simulink model "comprez"  (R2021b)
settings: Solver=VariableStepAuto  StartTime=0.0  StopTime=220  RelTol=1e-3
values from neighbouring files (symbols this model uses):
  AirDensity_kgpm3 = 1.225    [vehicle_controller.mat]
  BatteryCapacity_Wh = 83    [vehicle_controller.mat]
  BatteryInitialEnergy = 58.1    [vehicle_controller.mat]
  BatteryMaxVoltage_V = 96    [vehicle_controller.mat]
  BatteryVoltageCoefficient_x = [0 0.1 0.2 0.3 0.4 0.5 0.6 0.7 0.8 0.9 1]    [vehicle_controller.mat]
  BatteryVoltageCoefficient_y = [0.833333333333 0.85 0.866666666667 0.883333333333 0.9 0.916666666667 0.933333333333 0.95 0.966666666667 0.983333333333 1]    [vehicle_controller.mat]
  BodyInitialSpeed_mps = 0    [vehicle_controller.mat]
  BodyMass_kg = 900    [vehicle_controller.mat]
  CombustionEngineMaxTorque_Nm = 100    [vehicle_controller.mat]
  DragArea_m2 = 4.5    [vehicle_controller.mat]
  DragCoeficient_1 = 0.4    [vehicle_controller.mat]
  FrictionCoefficient_Nsprad = 0.01    [vehicle_controller.mat]
  GearboxRatio_0_1 = 3    [vehicle_controller.mat]
  Ke = 0.1178    [vehicle_controller.mat]
  Kt = 0.668    [vehicle_controller.mat]
  L = looptransfer.Lo    [H_infinity_control_design.m]    (also in LoopShaping.m = G*K; Vehicle_Car_Controller.m = P * C)
  R = 0.141176    [vehicle_controller.mat]
  WheelDiameter_m = 0.5    [vehicle_controller.mat]
undefined symbols (not defined in the file or in its folder): K
libraries: simulink x10, simulink_extras x3, neural x1
settings Model: Creator=beni  LastModifiedBy=beni

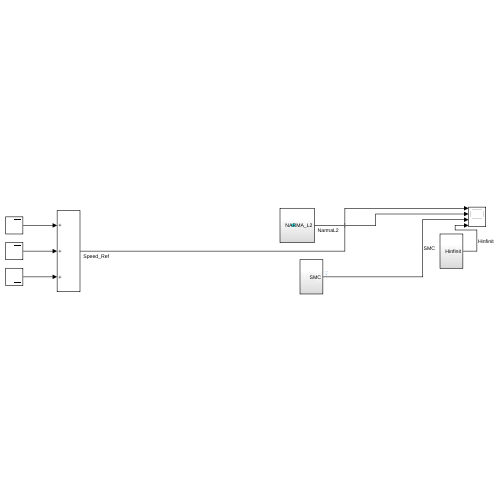
[thumbnail: Simulink's stored preview of the top-level diagram]
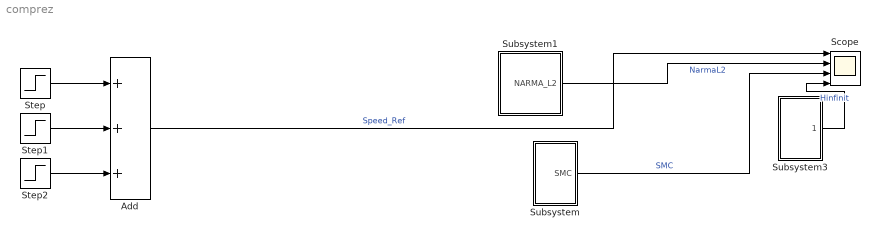
== system comprez ==
  Add : Sum  Inputs=+++
  Scope : Scope  NumInputPorts=4
  Step : Step  After=63  SampleTime=0
  Step1 : Step  Time=100  After=75  SampleTime=0
  Step2 : Step  Time=150  After=-20  SampleTime=0
  Subsystem : Subsystem
  Subsystem1 : Subsystem
  Subsystem3 : Subsystem
  wires:
  Subsystem1/1(NARMA_L2) -> Scope/2  "NarmaL2"
  Subsystem/1(SMC) -> Scope/3  "SMC"
  Subsystem3/1(Hinfinit) -> Scope/4  "Hinfinit"
  Step/1 -> Add/1
  Step2/1 -> Add/3
  Step1/1 -> Add/2
  Add/1 -> Scope/1  "Speed_Ref"

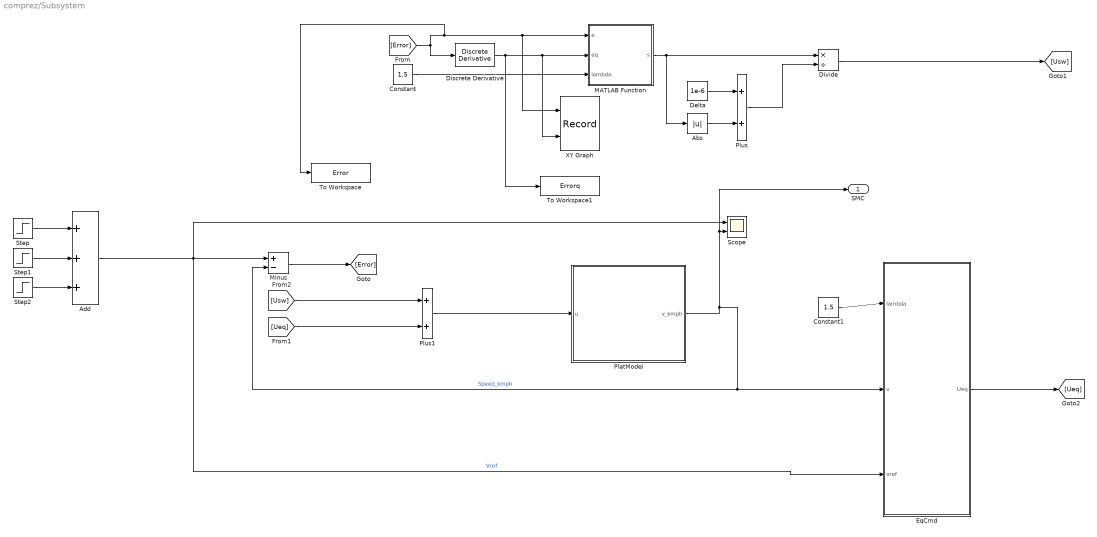
== system comprez/Subsystem ==
  Abs : Abs
  Add : Sum  Inputs=+++
  Constant : Constant  Value=1.5
  Constant1 : Constant  Value=1.5
  Delta : Constant  Value=1e-6
  Discrete Derivative : simulink/Discrete/Discrete Derivative  gainval=1.0  ICPrevScaledInput=0.0  OutMin=[]  OutMax=[]  OutDataType=fixdt(1, 16)  OutScaling=2^-10  DoSatur=off
  Divide : Product  Inputs=*/
  EqCmd : Subsystem
  MATLAB Function : MATLAB Function  TreatAsAtomicUnit=on
  Minus : Sum  Inputs=+-
  PlatModel : Subsystem
  Plus : Sum
  Plus1 : Sum
  Scope : Scope  NumInputPorts=2
  Step : Step  After=63  SampleTime=0
  Step1 : Step  Time=100  After=75  SampleTime=0
  Step2 : Step  Time=150  After=-20  SampleTime=0
  To Workspace : ToWorkspace  VariableName=Error  SampleTime=-1
  To Workspace1 : ToWorkspace  VariableName=Errorq  SampleTime=-1
  XY Graph : Record  FileSettingsInternal="{\"entries\":[{\"content\":{\"excelSettings\":{\"content\":{},\"type\":\"Streamout.ExcelSettings\"}},\"type\":\"Streamout.FileSettingStorage\",\"uuid\":\"431da7f9-c04b-4948-b4ed-e4a663989407\"}],\"packageUris\":[\"http://schema.mathworks.com/mf0/streamout_blocks/R2020a\"],\"version\":\"1.0\"}"  Layout=[1 1]  SignalsInternal="{\"entries\":[{\"content\":{\"signals\":[{\"content\":{\"blockPath\":[\"untitled/Subsystem/XY Graph\"],\"channel\":[],\"dimensions\":[1],\"domain\":\"untitled/Subsystem/XY Graph\",\"lineColor\":\"#77ac30\",\"plots\":[],\"port\":1,\"sid\":[\"\"],\"signalID\":461,\"signalName\":\"From\"},\"type\":\"RecordBlkView.Signal\",\"uuid\":\"f59c2270-2e51-4f55-abe7-1d4243515257\"},{\"content\":{\"blockPath\":[\"untitled/Subsystem/XY Graph\"],\"channel\":[],\"dimensions\":[1],\"domain\":\"untitled/Subsystem/XY Graph\",\"lineColor\":\"#4dbeee\",\"plots\":[],\"port\":2,\"sid\":[\"\"],\"signalID\":465,\"signalName\":\"Discrete Derivative\"},\"type\":\"RecordBlkView.Signal\",\"uuid\":\"50d11027-a391-472c-89af-c25c5bda5fe9\"}]},\"type\":\"RecordBlkView.InputSignals\",\"uuid\":\"2de3fad6-2ef4-449e-85cd-74187c4d7911\"}],\"packageUris\":[\"http://schema.mathworks.com/mf0/streamout_blocks/R2020a\"],\"version\":\"1.0\"}"  VisualizationBindings="{\"xyplotplugin\":{\"info\":[{\"series\":[],\"subplotID\":1}]}}"  CompatibilityTag=XY
  SMC : Outport
  wires:
  Delta/1 -> Plus/1
  EqCmd/1(Ueq) -> [Ueq]
  Constant/1 -> MATLAB Function/3(lambda)
  Step2/1 -> Add/3
  Discrete Derivative/1 -> To Workspace1/1, XY Graph/2, MATLAB Function/2(eq)
  Divide/1 -> [Usw]
  Plus1/1 -> PlatModel/1(u)
  [Error] -> Discrete Derivative/1, To Workspace/1, XY Graph/1, MATLAB Function/1(e)
  Constant1/1 -> EqCmd/1(lambda)
  Step1/1 -> Add/2
  PlatModel/1(v_kmph) -> SMC/1, Scope/2, Minus/2, EqCmd/2(v)  "Speed_kmph"
  [Ueq] -> Plus1/2
  MATLAB Function/1(s) -> Divide/1, Abs/1
  Minus/1 -> [Error]
  Add/1 -> Scope/1, EqCmd/3(vref), Minus/1  "Vref"
  [Usw] -> Plus1/1
  Step/1 -> Add/1
  Abs/1 -> Plus/2
  Plus/1 -> Divide/2

== system comprez/Subsystem1 ==
  Add : Sum  Inputs=+++
  NARMA-L2 Controller : neural/Control Systems/NARMA-L2 Controller  Normalize=0  IW1_1=[14.805701745740947217 14.646781356170984978 -2.6795517638832206941 -3.0429665609145888361;0.0082504465043554964243 -0.0031047596973149470083 -0.19104579150759948281 -0.0019065831191643792079;7.5749920141026407805 7.5802491884089882035 2.5258130278732027207 5.2003399921720587784;5.6443464414619350933 5.5593743114347526912 5.4574529164140681559 -1.262646873991036367;-0.077113742349454575398 -0.12421249851503408934 0.27616115965566950807 -3.0335571846180888755;1.3687979141489454715 1.348758547794491669 1.8430382789363553009 -4.4821808874517108379;7.4648043867614859437 6.9138040370909790155 -6.4521842638915769541 -6.4752629879810035263;0.25415811051558578892 0.27095489415654944176 0.33085125399628528831 -5.1587607384097351471;0.73490417335290436629 0.71397202774130674729 -2.7944141460391684895 -2.1433829785686704383;12.313347392571362349 12.290885057018957838 4.9134480385467735886 4.1442540648070789189]  IW3_2=[-0.53446907211207028698 -0.56584926038284277805 2.4772120111943900511 -3.9548848078019669394;-0.17438807197240477342 -0.22128333125178542562 1.5531169507607898161 -0.34520678882552874311;0.95091689639915899512 0.95028272165322946741 0.22539553833304259989 1.7331390891255484821;3.700630947998471143 3.7425256407849083473 -1.8851418393007957075 -2.2708954055355921042;0.88065998535395761948 0.88365446864527419368 1.5291495768605958272 2.4005012696654319804;-2.4137283268318223683 -2.4494453076346633935 -4.9927757014470763863 0.76018418227054873615;25.351825374508759836 25.27888711602448879 -4.7413628925274950987 -0.67383771249038093565;0.23168479727832039239 0.23277992322472923492 -4.1106914579192617154 -1.9950979166110411889;1.0386917909126904824 1.0340729140030018307 4.3711584253374500264 2.4067831249123865511;-0.38804355351227276527 -0.38312881003881188446 4.6834752181205132615 3.9688368481856413084]  IW5_3=6.3379737560603359725  LW2_1=[-12.476146884958998484 20.132559713911909682 1.2837858310253040806 0.47110125335549535297 -3.4715679157995884552 1.5639086465487934685 -9.1062933601963358399 2.2538229413428849668 1.1799476813699860678 15.006187931304040717]  LW4_3=[1.1330197318124872741 -0.32308713263636479329 0.38063538092662579926 -0.99546710331545062989 -0.43691353799223309196 1.4840354658163856794 -0.49171464039683382419 -0.86552916277619362795 -0.45557558379852736152 -0.41489442559775752128]  LW5_4=-1.0550086150086563919  LW6_5=1.0150981461816406259  LW6_2=9.4619394816672333093  B1=[7.4080490716640348126;-0.36234293340332640598;-1.2825203054346920872;0.27247158620995243217;-1.6827356510965316705;2.9673472765957158437;-16.208928034510176275;1.9238958992426151706;3.5334077697743180302;-1.7925756402558468139]  B2=3.7495520554947892045  B3=[-0.26350487256121968294;-2.6083435985723815165;3.8381459366534440569;3.6501032408282689801;1.4758419519326404501;2.8923530689336272026;5.3210473908125628384;4.2017271567726295345;-3.5443507400312395106;-3.0836228084886676548]  B4=-1.0103082685048965228  Limit_output=1  min_output=0  max_output=250  Use_Previous_Weights=1  Ts=0.01  S1=10  Ni=3  Nj=2  sim_file=Car_Plant  trainfun=trainlm  Use_validation=1  Use_Testing=1  max_i=0.9  min_i=0.1  max_i_int=10  min_i_int=5  sam_training=10000  epochs=4000  minp=0.10041790028555581948  maxp=0.89926431580908861019  mint=0  maxt=0.89926431580908861019
      settings: SourceProductBaseCode=NN
  Step : Step  After=63  SampleTime=0
  Step1 : Step  Time=100  After=75  SampleTime=0
  Step2 : Step  Time=150  After=-20  SampleTime=0
  Subsystem : Subsystem
  NARMA_L2 : Outport
  wires:
  Step/1 -> Add/1
  NARMA-L2 Controller/1 -> Subsystem/1(DutyCycle_1)
  Step1/1 -> Add/2
  Subsystem/1(VechicleSpeed_kmph) -> NARMA_L2/1, NARMA-L2 Controller/2  "Speed_Kmph"
  Add/1 -> NARMA-L2 Controller/1  "Speed_Ref"
  Step2/1 -> Add/3

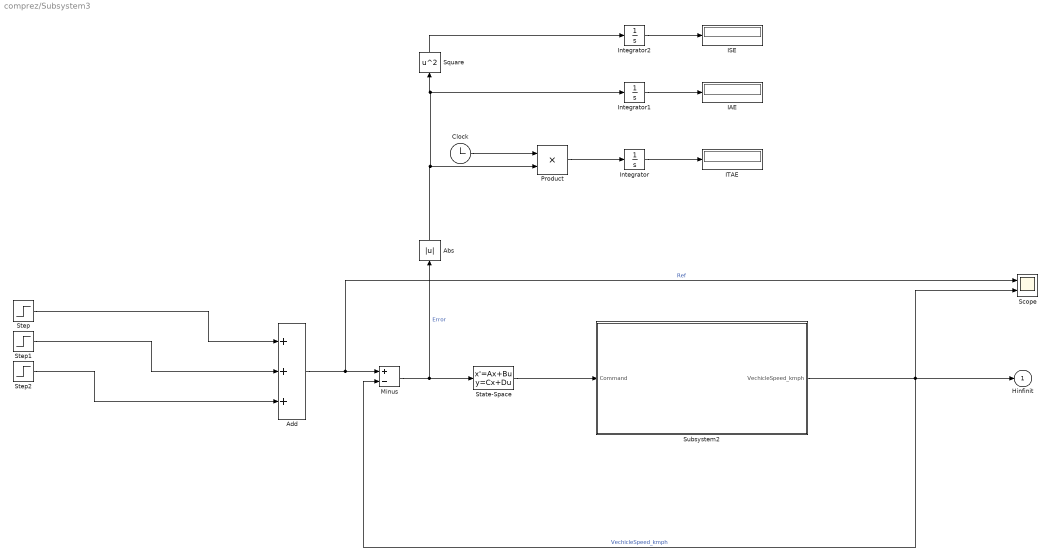
== system comprez/Subsystem3 ==
  Abs : Abs
  Add : Sum  Inputs=+++
  Clock : Clock
  IAE : Display
  ISE : Display
  ITAE : Display
  Integrator : Integrator
  Integrator1 : Integrator
  Integrator2 : Integrator
  Minus : Sum  Inputs=+-
  Product : Product
  Scope : Scope  NumInputPorts=2
  Square : Math  Operator=square  SaturateOnIntegerOverflow=on
  State-Space : StateSpace  A=K.A  B=K.B  C=K.C  D=K.D  InitialCondition=0
  Step : Step  After=63  SampleTime=0
  Step1 : Step  Time=100  After=75  SampleTime=0
  Step2 : Step  Time=150  After=-20  SampleTime=0
  Subsystem2 : Subsystem
  Hinfinit : Outport
  wires:
  Square/1 -> Integrator2/1
  Integrator1/1 -> IAE/1
  State-Space/1 -> Subsystem2/1(Command)
  Product/1 -> Integrator/1
  Add/1 -> Scope/1, Minus/1  "Ref"
  Integrator2/1 -> ISE/1
  Subsystem2/1(VechicleSpeed_kmph) -> Hinfinit/1, Scope/2, Minus/2  "VechicleSpeed_kmph"
  Step1/1 -> Add/2
  Step/1 -> Add/1
  Abs/1 -> Square/1, Integrator1/1, Product/2
  Step2/1 -> Add/3
  Minus/1 -> Abs/1, State-Space/1  "Error"
  Clock/1 -> Product/1
  Integrator/1 -> ITAE/1

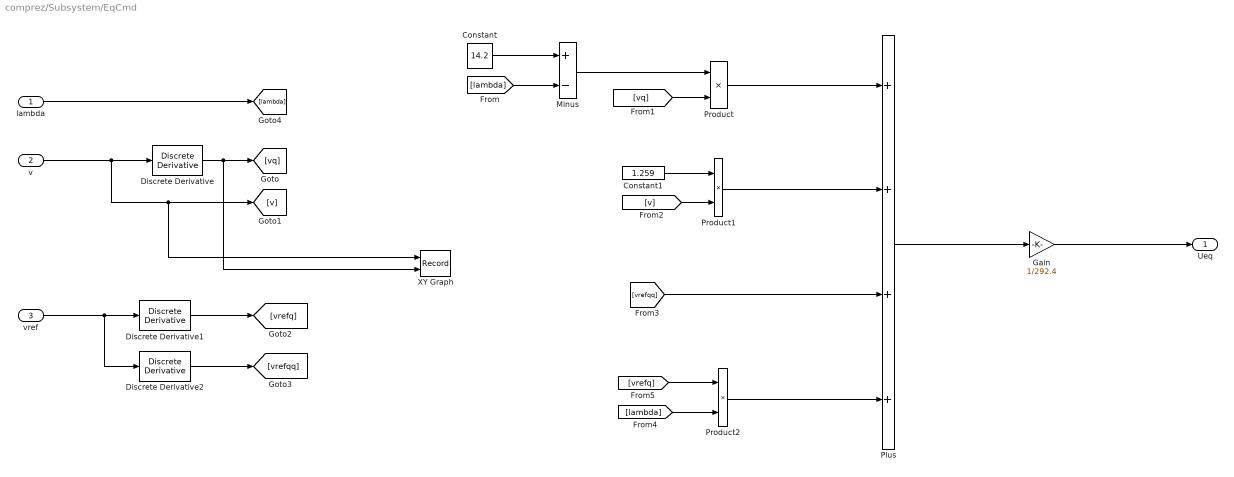
== system comprez/Subsystem/EqCmd ==
  lambda : Inport
  v : Inport  Port=2
  vref : Inport  Port=3
  Constant : Constant  Value=14.2
  Constant1 : Constant  Value=1.259
  Discrete Derivative : simulink/Discrete/Discrete Derivative  gainval=1.0  ICPrevScaledInput=0.0  OutMin=[]  OutMax=[]  OutDataType=fixdt(1, 16)  OutScaling=2^-10  DoSatur=off
  Discrete Derivative1 : simulink/Discrete/Discrete Derivative  gainval=1.0  ICPrevScaledInput=0.0  OutMin=[]  OutMax=[]  OutDataType=fixdt(1, 16)  OutScaling=2^-10  DoSatur=off
  Discrete Derivative2 : simulink/Discrete/Discrete Derivative  gainval=1.0  ICPrevScaledInput=0.0  OutMin=[]  OutMax=[]  OutDataType=fixdt(1, 16)  OutScaling=2^-10  DoSatur=off
  Gain : Gain  Gain=1/292.4
  Minus : Sum  Inputs=+-
  Plus : Sum  Inputs=++++
  Product : Product
  Product1 : Product
  Product2 : Product
  XY Graph : Record  FileSettingsInternal="{\"entries\":[{\"content\":{\"excelSettings\":{\"content\":{},\"type\":\"Streamout.ExcelSettings\"}},\"type\":\"Streamout.FileSettingStorage\",\"uuid\":\"307b3435-70e1-4ce0-9e61-10e40ea3230f\"}],\"packageUris\":[\"http://schema.mathworks.com/mf0/streamout_blocks/R2020a\"],\"version\":\"1.0\"}"  Layout=[1 1]  SignalsInternal="{\"entries\":[{\"content\":{\"signals\":[{\"content\":{\"blockPath\":[\"untitled/Subsystem/EqCmd/XY Graph\"],\"channel\":[],\"dimensions\":[1],\"domain\":\"untitled/Subsystem/EqCmd/XY Graph\",\"lineColor\":\"#ff6929\",\"plots\":[],\"port\":1,\"sid\":[\"\"],\"signalID\":477,\"signalName\":\"v\"},\"type\":\"RecordBlkView.Signal\",\"uuid\":\"07e0db4b-b093-4305-a7e8-4611508c29d2\"},{\"content\":{\"blockPath\":[\"untitled/Subsystem/EqCmd/XY Graph\"],\"channel\":[],\"dimensions\":[1],\"domain\":\"untitled/Subsystem/EqCmd/XY Graph\",\"lineColor\":\"#b746ff\",\"plots\":[],\"port\":2,\"sid\":[\"\"],\"signalID\":481,\"signalName\":\"Discrete Derivative\"},\"type\":\"RecordBlkView.Signal\",\"uuid\":\"dc14ac50-79be-4a5f-948c-baa6f1a01df7\"}]},\"type\":\"RecordBlkView.InputSignals\",\"uuid\":\"5ada03a2-bf2c-4373-b1b1-8d91b22b2de5\"}],\"packageUris\":[\"http://schema.mathworks.com/mf0/streamout_blocks/R2020a\"],\"version\":\"1.0\"}"  VisualizationBindings="{\"xyplotplugin\":{\"info\":[{\"series\":[],\"subplotID\":1}]}}"  CompatibilityTag=XY
  Ueq : Outport
  wires:
  v/1 -> Discrete Derivative/1, XY Graph/1, [v]
  Discrete Derivative/1 -> XY Graph/2, [vq]
  vref/1 -> Discrete Derivative2/1, Discrete Derivative1/1
  Discrete Derivative1/1 -> [vrefq]
  Discrete Derivative2/1 -> [vrefqq]
  lambda/1 -> [lambda]
  Constant/1 -> Minus/1
  [lambda] -> Minus/2
  Minus/1 -> Product/1
  [vq] -> Product/2
  Product/1 -> Plus/1
  Constant1/1 -> Product1/1
  [v] -> Product1/2
  Product1/1 -> Plus/2
  [vrefqq] -> Plus/3
  Product2/1 -> Plus/4
  [lambda] -> Product2/2
  [vrefq] -> Product2/1
  Plus/1 -> Gain/1
  Gain/1 -> Ueq/1

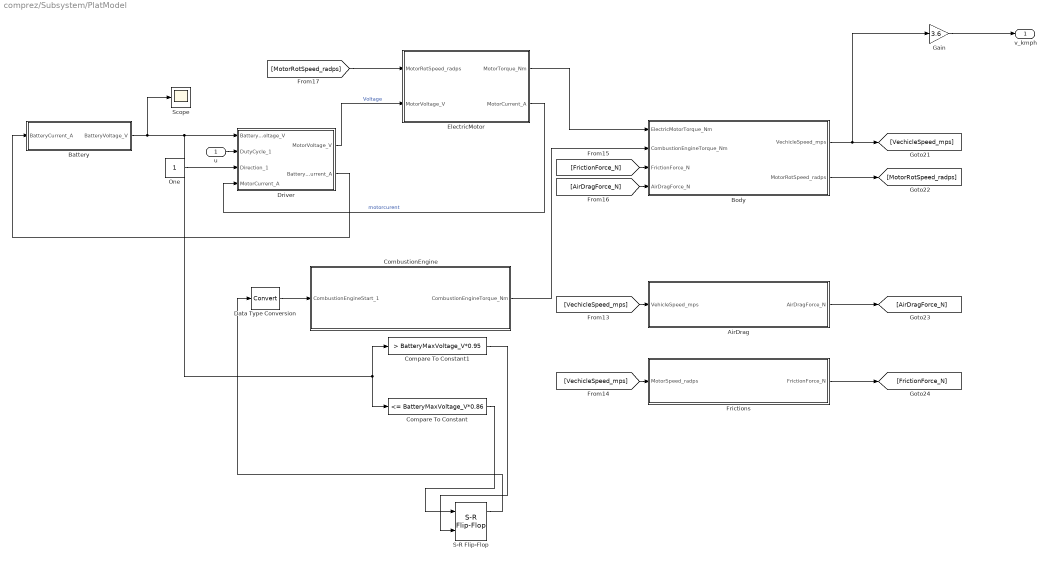
== system comprez/Subsystem/PlatModel ==
  u : Inport
  AirDrag : Subsystem
  Battery : Subsystem
  Body : Subsystem
  CombustionEngine : Subsystem
  Compare To Constant : simulink/Logic and Bit Operations/Compare To Constant  relop=<=  const=BatteryMaxVoltage_V*0.86  OutDataTypeStr=boolean
  Compare To Constant1 : simulink/Logic and Bit Operations/Compare To Constant  relop=>  const=BatteryMaxVoltage_V*0.95  OutDataTypeStr=boolean
  Data Type Conversion : DataTypeConversion
  Driver : Subsystem
  ElectricMotor : Subsystem
  Frictions : Subsystem
  Gain : Gain  Gain=3.6
  One : Constant  OutDataTypeStr=Inherit: Inherit via back propagation
  S-R Flip-Flop : simulink_extras/Flip Flops/S-R Flip-Flop  initial_condition=0
  Scope : Scope
  v_kmph : Outport
  wires:
  One/1 -> Driver/3(Direction_1)
  ElectricMotor/1(MotorTorque_Nm) -> Body/1(ElectricMotorTorque_Nm)
  [FrictionForce_N] -> Body/3(FrictionForce_N)
  Body/1(VechicleSpeed_mps) -> [VechicleSpeed_mps], Gain/1
  Body/2(MotorRotSpeed_radps) -> [MotorRotSpeed_radps]
  AirDrag/1(AirDragForce_N) -> [AirDragForce_N]
  Frictions/1(FrictionForce_N) -> [FrictionForce_N]
  [VechicleSpeed_mps] -> AirDrag/1(VehicleSpeed_mps)
  [AirDragForce_N] -> Body/4(AirDragForce_N)
  [MotorRotSpeed_radps] -> ElectricMotor/1(MotorRotSpeed_radps)
  [VechicleSpeed_mps] -> Frictions/1(MotorSpeed_radps)
  ElectricMotor/2(MotorCurrent_A) -> Driver/4(MotorCurrent_A)  "motorcurent"
  u/1 -> Driver/2(DutyCycle_1)
  Gain/1 -> v_kmph/1
  Data Type Conversion/1 -> CombustionEngine/1(CombustionEngineStart_1)
  CombustionEngine/1(CombustionEngineTorque_Nm) -> Body/2(CombustionEngineTorque_Nm)
  Driver/2(BatteryCurrent_A) -> Battery/1(BatteryCurrent_A)
  Driver/1(MotorVoltage_V) -> ElectricMotor/2(MotorVoltage_V)  "Voltage"
  Compare To Constant1/1 -> S-R Flip-Flop/2
  Compare To Constant/1 -> S-R Flip-Flop/1
  S-R Flip-Flop/1 -> Data Type Conversion/1
  Battery/1(BatteryVoltage_V) -> Scope/1, Driver/1(BatteryVoltage_V), Compare To Constant1/1, Compare To Constant/1

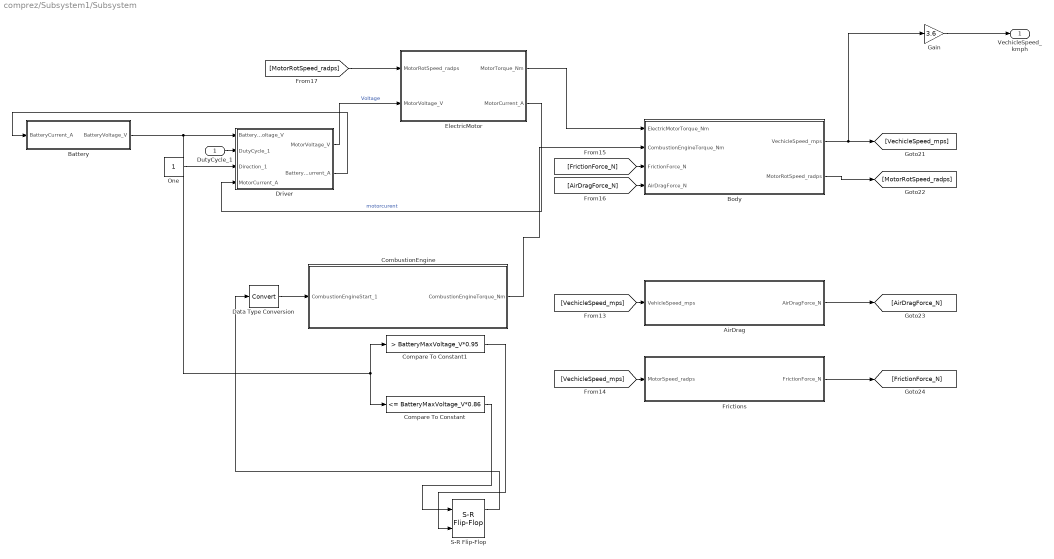
== system comprez/Subsystem1/Subsystem ==
  DutyCycle_1 : Inport
  AirDrag : Subsystem
  Battery : Subsystem
  Body : Subsystem
  CombustionEngine : Subsystem
  Compare To Constant : simulink/Logic and Bit Operations/Compare To Constant  relop=<=  const=BatteryMaxVoltage_V*0.86  OutDataTypeStr=boolean
  Compare To Constant1 : simulink/Logic and Bit Operations/Compare To Constant  relop=>  const=BatteryMaxVoltage_V*0.95  OutDataTypeStr=boolean
  Data Type Conversion : DataTypeConversion
  Driver : Subsystem
  ElectricMotor : Subsystem
  Frictions : Subsystem
  Gain : Gain  Gain=3.6
  One : Constant  OutDataTypeStr=Inherit: Inherit via back propagation
  S-R Flip-Flop : simulink_extras/Flip Flops/S-R Flip-Flop  initial_condition=0
  VechicleSpeed_kmph : Outport
  wires:
  One/1 -> Driver/3(Direction_1)
  ElectricMotor/1(MotorTorque_Nm) -> Body/1(ElectricMotorTorque_Nm)
  [FrictionForce_N] -> Body/3(FrictionForce_N)
  Body/1(VechicleSpeed_mps) -> [VechicleSpeed_mps], Gain/1
  Body/2(MotorRotSpeed_radps) -> [MotorRotSpeed_radps]
  AirDrag/1(AirDragForce_N) -> [AirDragForce_N]
  Frictions/1(FrictionForce_N) -> [FrictionForce_N]
  [VechicleSpeed_mps] -> AirDrag/1(VehicleSpeed_mps)
  [AirDragForce_N] -> Body/4(AirDragForce_N)
  [MotorRotSpeed_radps] -> ElectricMotor/1(MotorRotSpeed_radps)
  [VechicleSpeed_mps] -> Frictions/1(MotorSpeed_radps)
  ElectricMotor/2(MotorCurrent_A) -> Driver/4(MotorCurrent_A)  "motorcurent"
  DutyCycle_1/1 -> Driver/2(DutyCycle_1)
  Gain/1 -> VechicleSpeed_kmph/1
  Data Type Conversion/1 -> CombustionEngine/1(CombustionEngineStart_1)
  CombustionEngine/1(CombustionEngineTorque_Nm) -> Body/2(CombustionEngineTorque_Nm)
  Driver/2(BatteryCurrent_A) -> Battery/1(BatteryCurrent_A)
  Driver/1(MotorVoltage_V) -> ElectricMotor/2(MotorVoltage_V)  "Voltage"
  Compare To Constant1/1 -> S-R Flip-Flop/2
  Compare To Constant/1 -> S-R Flip-Flop/1
  S-R Flip-Flop/1 -> Data Type Conversion/1
  Battery/1(BatteryVoltage_V) -> Driver/1(BatteryVoltage_V), Compare To Constant1/1, Compare To Constant/1

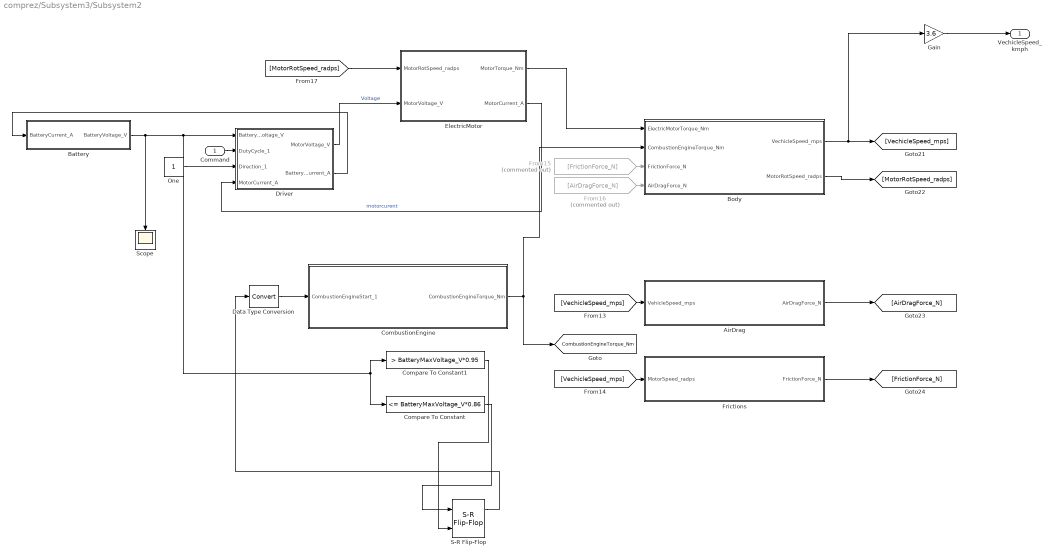
== system comprez/Subsystem3/Subsystem2 ==
  Command : Inport
  AirDrag : Subsystem
  Battery : Subsystem
  Body : Subsystem
  CombustionEngine : Subsystem
  Compare To Constant : simulink/Logic and Bit Operations/Compare To Constant  relop=<=  const=BatteryMaxVoltage_V*0.86  OutDataTypeStr=boolean
  Compare To Constant1 : simulink/Logic and Bit Operations/Compare To Constant  relop=>  const=BatteryMaxVoltage_V*0.95  OutDataTypeStr=boolean
  Data Type Conversion : DataTypeConversion
  Driver : Subsystem
  ElectricMotor : Subsystem
  Frictions : Subsystem
  From15 : From  Commented=on  GotoTag=FrictionForce_N
  From16 : From  Commented=on  GotoTag=AirDragForce_N
  Gain : Gain  Gain=3.6
  One : Constant  OutDataTypeStr=Inherit: Inherit via back propagation
  S-R Flip-Flop : simulink_extras/Flip Flops/S-R Flip-Flop  initial_condition=0
  Scope : Scope
  VechicleSpeed_kmph : Outport
  tag scope: CombustionEngineTorque_Nm=global
  wires:
  One/1 -> Driver/3(Direction_1)
  ElectricMotor/1(MotorTorque_Nm) -> Body/1(ElectricMotorTorque_Nm)
  From15/1 -> Body/3(FrictionForce_N)
  Body/1(VechicleSpeed_mps) -> [VechicleSpeed_mps], Gain/1
  Body/2(MotorRotSpeed_radps) -> [MotorRotSpeed_radps]
  AirDrag/1(AirDragForce_N) -> [AirDragForce_N]
  Frictions/1(FrictionForce_N) -> [FrictionForce_N]
  [VechicleSpeed_mps] -> AirDrag/1(VehicleSpeed_mps)
  From16/1 -> Body/4(AirDragForce_N)
  [MotorRotSpeed_radps] -> ElectricMotor/1(MotorRotSpeed_radps)
  [VechicleSpeed_mps] -> Frictions/1(MotorSpeed_radps)
  ElectricMotor/2(MotorCurrent_A) -> Driver/4(MotorCurrent_A)  "motorcurent"
  Command/1 -> Driver/2(DutyCycle_1)
  Gain/1 -> VechicleSpeed_kmph/1
  Data Type Conversion/1 -> CombustionEngine/1(CombustionEngineStart_1)
  CombustionEngine/1(CombustionEngineTorque_Nm) -> Body/2(CombustionEngineTorque_Nm), [CombustionEngineTorque_Nm]
  Driver/2(BatteryCurrent_A) -> Battery/1(BatteryCurrent_A)
  Driver/1(MotorVoltage_V) -> ElectricMotor/2(MotorVoltage_V)  "Voltage"
  Compare To Constant1/1 -> S-R Flip-Flop/2
  Compare To Constant/1 -> S-R Flip-Flop/1
  S-R Flip-Flop/1 -> Data Type Conversion/1
  Battery/1(BatteryVoltage_V) -> Scope/1, Driver/1(BatteryVoltage_V), Compare To Constant1/1, Compare To Constant/1

== system comprez/Subsystem/PlatModel/AirDrag ==
  VehicleSpeed_mps : Inport
  " " : Constant  Value=0.5
  AirDensity_kgpm3 : Constant  Value=AirDensity_kgpm3
  DragArea_m2 : Constant  Value=DragArea_m2
  DragCoeficient_1 : Constant  Value=DragCoeficient_1
  Product : Product  Inputs=5
  Square : Math  Operator=square  SaturateOnIntegerOverflow=on
  AirDragForce_N : Outport
  wires:
  VehicleSpeed_mps/1 -> Square/1
  Square/1 -> Product/5
  DragArea_m2/1 -> Product/3
  AirDensity_kgpm3/1 -> Product/4
  DragCoeficient_1/1 -> Product/2
  " "/1 -> Product/1
  Product/1 -> AirDragForce_N/1

== system comprez/Subsystem/PlatModel/Battery ==
  BatteryCurrent_A : Inport
  1-D Lookup Table : Lookup_n-D  NumberOfTableDimensions=1  BreakpointsForDimension1=BatteryVoltageCoefficient_x  Table=BatteryVoltageCoefficient_y  InternalRulePriority=Speed  RndMeth=Simplest  InputSameDT=on
  BatteryCapacity_Wh : Constant  Value=BatteryCapacity_Wh
  BatteryMaxVoltage_V : Constant  Value=BatteryMaxVoltage_V
  Gain : Gain  Gain=-1
  Gain1 : Gain  Gain=1/3600
  Integrator : Integrator  InitialCondition=BatteryInitialEnergy
  Product : Product
  Product1 : Product  Inputs=*/
  Product2 : Product
  BatteryVoltage_V : Outport
  wires:
  BatteryCurrent_A/1 -> Product2/1  "BatteryCurrent_A"
  Product/1 -> Product2/2, BatteryVoltage_V/1  "BatteryVoltage_V"
  Integrator/1 -> Product1/1  "Energy_Wh"
  1-D Lookup Table/1 -> Product/2  "VoltageCoeficient_0_1"
  BatteryMaxVoltage_V/1 -> Product/1
  BatteryCapacity_Wh/1 -> Product1/2
  Product1/1 -> 1-D Lookup Table/1  "StateOfCharge_0_1"
  Product2/1 -> Gain/1
  Gain/1 -> Gain1/1
  Gain1/1 -> Integrator/1

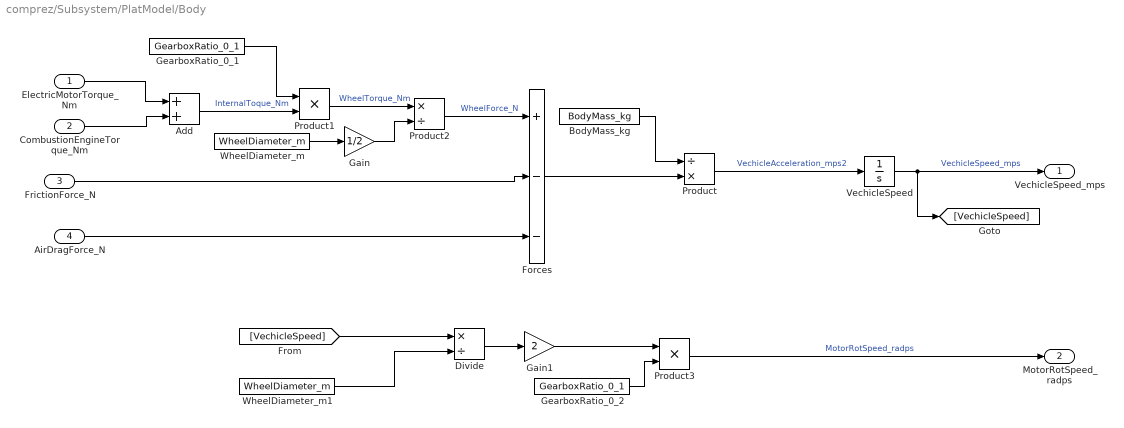
== system comprez/Subsystem/PlatModel/Body ==
  ElectricMotorTorque_Nm : Inport
  CombustionEngineTorque_Nm : Inport  Port=2
  FrictionForce_N : Inport  Port=3
  AirDragForce_N : Inport  Port=4
  Add : Sum
  BodyMass_kg : Constant  Value=BodyMass_kg
  Divide : Product  Inputs=*/
  Forces : Sum  Inputs=+--
  Gain : Gain  Gain=1/2
  Gain1 : Gain  Gain=2
  GearboxRatio_0_1 : Constant  Value=GearboxRatio_0_1
  GearboxRatio_0_2 : Constant  Value=GearboxRatio_0_1
  Product : Product  Inputs=/*
  Product1 : Product
  Product2 : Product  Inputs=*/
  Product3 : Product  Inputs=**
  VechicleSpeed : Integrator  InitialCondition=BodyInitialSpeed_mps
  WheelDiameter_m : Constant  Value=WheelDiameter_m
  WheelDiameter_m1 : Constant  Value=WheelDiameter_m
  VechicleSpeed_mps : Outport
  MotorRotSpeed_radps : Outport  Port=2
  wires:
  VechicleSpeed/1 -> [VechicleSpeed], VechicleSpeed_mps/1  "VechicleSpeed_mps"
  Product/1 -> VechicleSpeed/1  "VechicleAcceleration_mps2"
  BodyMass_kg/1 -> Product/1
  Forces/1 -> Product/2
  AirDragForce_N/1 -> Forces/3
  FrictionForce_N/1 -> Forces/2
  ElectricMotorTorque_Nm/1 -> Add/1
  CombustionEngineTorque_Nm/1 -> Add/2
  Add/1 -> Product1/2  "InternalToque_Nm"
  GearboxRatio_0_1/1 -> Product1/1
  Product1/1 -> Product2/1  "WheelTorque_Nm"
  WheelDiameter_m/1 -> Gain/1
  Product2/1 -> Forces/1  "WheelForce_N"
  Gain/1 -> Product2/2
  [VechicleSpeed] -> Divide/1
  WheelDiameter_m1/1 -> Divide/2
  Divide/1 -> Gain1/1
  Gain1/1 -> Product3/1
  GearboxRatio_0_2/1 -> Product3/2
  Product3/1 -> MotorRotSpeed_radps/1  "MotorRotSpeed_radps"

== system comprez/Subsystem/PlatModel/CombustionEngine ==
  CombustionEngineStart_1 : Inport
  Gain : Gain  Gain=CombustionEngineMaxTorque_Nm
  Transfer Fcn : TransferFcn  Denominator=[1 1]
  CombustionEngineTorque_Nm : Outport
  wires:
  Transfer Fcn/1 -> CombustionEngineTorque_Nm/1
  CombustionEngineStart_1/1 -> Gain/1
  Gain/1 -> Transfer Fcn/1

== system comprez/Subsystem/PlatModel/Driver ==
  BatteryVoltage_V : Inport
  DutyCycle_1 : Inport  Port=2
  Direction_1 : Inport  Port=3
  MotorCurrent_A : Inport  Port=4
  Product : Product
  Product1 : Product
  Product2 : Product
  MotorVoltage_V : Outport
  BatteryCurrent_A : Outport  Port=2
  wires:
  BatteryVoltage_V/1 -> Product/1
  Product/1 -> MotorVoltage_V/1
  Product2/1 -> Product1/1, Product/2
  MotorCurrent_A/1 -> Product1/2
  Product1/1 -> BatteryCurrent_A/1
  DutyCycle_1/1 -> Product2/1
  Direction_1/1 -> Product2/2

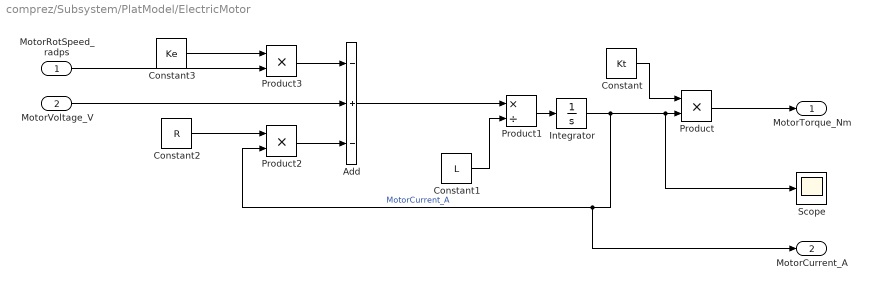
== system comprez/Subsystem/PlatModel/ElectricMotor ==
  MotorRotSpeed_radps : Inport
  MotorVoltage_V : Inport  Port=2
  Add : Sum  Inputs=-+-
  Constant : Constant  Value=Kt
  Constant1 : Constant  Value=L
  Constant2 : Constant  Value=R
  Constant3 : Constant  Value=Ke
  Integrator : Integrator
  Product : Product
  Product1 : Product  Inputs=*/
  Product2 : Product
  Product3 : Product
  Scope : Scope
  MotorTorque_Nm : Outport
  MotorCurrent_A : Outport  Port=2
  wires:
  Product/1 -> MotorTorque_Nm/1
  Integrator/1 -> MotorCurrent_A/1, Product2/2, Scope/1, Product/2  "MotorCurrent_A"
  Constant/1 -> Product/1
  Product1/1 -> Integrator/1
  Constant1/1 -> Product1/2
  Add/1 -> Product1/1
  Product2/1 -> Add/3
  Constant2/1 -> Product2/1
  MotorVoltage_V/1 -> Add/2
  Constant3/1 -> Product3/1
  Product3/1 -> Add/1
  MotorRotSpeed_radps/1 -> Product3/2

== system comprez/Subsystem/PlatModel/Frictions ==
  MotorSpeed_radps : Inport
  FrictionCoefficient_Nsprad : Constant  Value=FrictionCoefficient_Nsprad
  Product : Product
  FrictionForce_N : Outport
  wires:
  Product/1 -> FrictionForce_N/1
  MotorSpeed_radps/1 -> Product/2
  FrictionCoefficient_Nsprad/1 -> Product/1

== system comprez/Subsystem1/Subsystem/AirDrag ==
  VehicleSpeed_mps : Inport
  " " : Constant  Value=0.5
  AirDensity_kgpm3 : Constant  Value=AirDensity_kgpm3
  DragArea_m2 : Constant  Value=DragArea_m2
  DragCoeficient_1 : Constant  Value=DragCoeficient_1
  Product : Product  Inputs=5
  Square : Math  Operator=square  SaturateOnIntegerOverflow=on
  AirDragForce_N : Outport
  wires:
  VehicleSpeed_mps/1 -> Square/1
  Square/1 -> Product/5
  DragArea_m2/1 -> Product/3
  AirDensity_kgpm3/1 -> Product/4
  DragCoeficient_1/1 -> Product/2
  " "/1 -> Product/1
  Product/1 -> AirDragForce_N/1

== system comprez/Subsystem1/Subsystem/Battery ==
  BatteryCurrent_A : Inport
  1-D Lookup Table : Lookup_n-D  NumberOfTableDimensions=1  BreakpointsForDimension1=BatteryVoltageCoefficient_x  Table=BatteryVoltageCoefficient_y  InternalRulePriority=Speed  RndMeth=Simplest  InputSameDT=on
  BatteryCapacity_Wh : Constant  Value=BatteryCapacity_Wh
  BatteryMaxVoltage_V : Constant  Value=BatteryMaxVoltage_V
  Gain : Gain  Gain=-1
  Gain1 : Gain  Gain=1/3600
  Integrator : Integrator  InitialCondition=BatteryInitialEnergy
  Product : Product
  Product1 : Product  Inputs=*/
  Product2 : Product
  BatteryVoltage_V : Outport
  wires:
  BatteryCurrent_A/1 -> Product2/1  "BatteryCurrent_A"
  Product/1 -> Product2/2, BatteryVoltage_V/1  "BatteryVoltage_V"
  Integrator/1 -> Product1/1  "Energy_Wh"
  1-D Lookup Table/1 -> Product/2  "VoltageCoeficient_0_1"
  BatteryMaxVoltage_V/1 -> Product/1
  BatteryCapacity_Wh/1 -> Product1/2
  Product1/1 -> 1-D Lookup Table/1  "StateOfCharge_0_1"
  Product2/1 -> Gain/1
  Gain/1 -> Gain1/1
  Gain1/1 -> Integrator/1

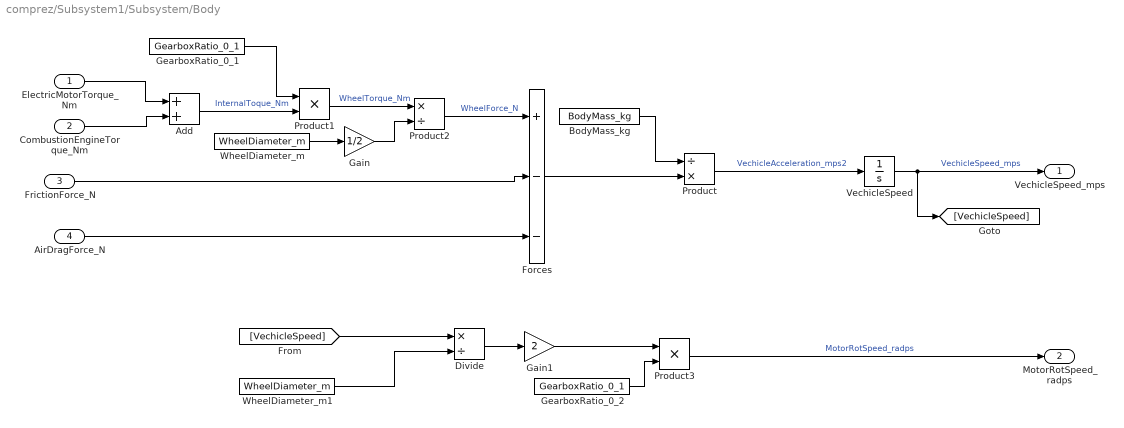
== system comprez/Subsystem1/Subsystem/Body ==
  ElectricMotorTorque_Nm : Inport
  CombustionEngineTorque_Nm : Inport  Port=2
  FrictionForce_N : Inport  Port=3
  AirDragForce_N : Inport  Port=4
  Add : Sum
  BodyMass_kg : Constant  Value=BodyMass_kg
  Divide : Product  Inputs=*/
  Forces : Sum  Inputs=+--
  Gain : Gain  Gain=1/2
  Gain1 : Gain  Gain=2
  GearboxRatio_0_1 : Constant  Value=GearboxRatio_0_1
  GearboxRatio_0_2 : Constant  Value=GearboxRatio_0_1
  Product : Product  Inputs=/*
  Product1 : Product
  Product2 : Product  Inputs=*/
  Product3 : Product  Inputs=**
  VechicleSpeed : Integrator  InitialCondition=BodyInitialSpeed_mps
  WheelDiameter_m : Constant  Value=WheelDiameter_m
  WheelDiameter_m1 : Constant  Value=WheelDiameter_m
  VechicleSpeed_mps : Outport
  MotorRotSpeed_radps : Outport  Port=2
  wires:
  VechicleSpeed/1 -> [VechicleSpeed], VechicleSpeed_mps/1  "VechicleSpeed_mps"
  Product/1 -> VechicleSpeed/1  "VechicleAcceleration_mps2"
  BodyMass_kg/1 -> Product/1
  Forces/1 -> Product/2
  AirDragForce_N/1 -> Forces/3
  FrictionForce_N/1 -> Forces/2
  ElectricMotorTorque_Nm/1 -> Add/1
  CombustionEngineTorque_Nm/1 -> Add/2
  Add/1 -> Product1/2  "InternalToque_Nm"
  GearboxRatio_0_1/1 -> Product1/1
  Product1/1 -> Product2/1  "WheelTorque_Nm"
  WheelDiameter_m/1 -> Gain/1
  Product2/1 -> Forces/1  "WheelForce_N"
  Gain/1 -> Product2/2
  [VechicleSpeed] -> Divide/1
  WheelDiameter_m1/1 -> Divide/2
  Divide/1 -> Gain1/1
  Gain1/1 -> Product3/1
  GearboxRatio_0_2/1 -> Product3/2
  Product3/1 -> MotorRotSpeed_radps/1  "MotorRotSpeed_radps"

== system comprez/Subsystem1/Subsystem/CombustionEngine ==
  CombustionEngineStart_1 : Inport
  Gain : Gain  Gain=CombustionEngineMaxTorque_Nm
  Transfer Fcn : TransferFcn  Denominator=[1 1]
  CombustionEngineTorque_Nm : Outport
  wires:
  Transfer Fcn/1 -> CombustionEngineTorque_Nm/1
  CombustionEngineStart_1/1 -> Gain/1
  Gain/1 -> Transfer Fcn/1

== system comprez/Subsystem1/Subsystem/Driver ==
  BatteryVoltage_V : Inport
  DutyCycle_1 : Inport  Port=2
  Direction_1 : Inport  Port=3
  MotorCurrent_A : Inport  Port=4
  Product : Product
  Product1 : Product
  Product2 : Product
  MotorVoltage_V : Outport
  BatteryCurrent_A : Outport  Port=2
  wires:
  BatteryVoltage_V/1 -> Product/1
  Product/1 -> MotorVoltage_V/1
  Product2/1 -> Product1/1, Product/2
  MotorCurrent_A/1 -> Product1/2
  Product1/1 -> BatteryCurrent_A/1
  DutyCycle_1/1 -> Product2/1
  Direction_1/1 -> Product2/2

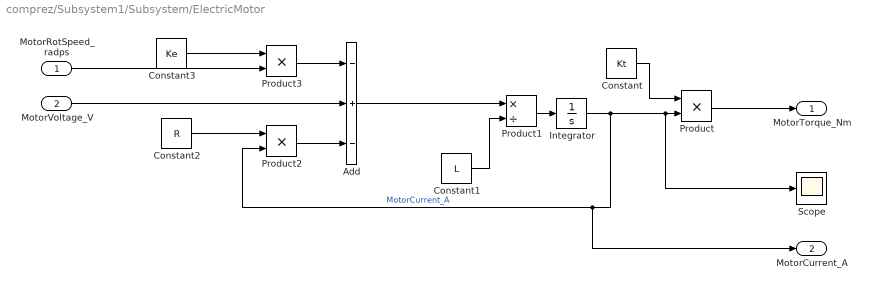
== system comprez/Subsystem1/Subsystem/ElectricMotor ==
  MotorRotSpeed_radps : Inport
  MotorVoltage_V : Inport  Port=2
  Add : Sum  Inputs=-+-
  Constant : Constant  Value=Kt
  Constant1 : Constant  Value=L
  Constant2 : Constant  Value=R
  Constant3 : Constant  Value=Ke
  Integrator : Integrator
  Product : Product
  Product1 : Product  Inputs=*/
  Product2 : Product
  Product3 : Product
  Scope : Scope
  MotorTorque_Nm : Outport
  MotorCurrent_A : Outport  Port=2
  wires:
  Product/1 -> MotorTorque_Nm/1
  Integrator/1 -> MotorCurrent_A/1, Product2/2, Scope/1, Product/2  "MotorCurrent_A"
  Constant/1 -> Product/1
  Product1/1 -> Integrator/1
  Constant1/1 -> Product1/2
  Add/1 -> Product1/1
  Product2/1 -> Add/3
  Constant2/1 -> Product2/1
  MotorVoltage_V/1 -> Add/2
  Constant3/1 -> Product3/1
  Product3/1 -> Add/1
  MotorRotSpeed_radps/1 -> Product3/2

== system comprez/Subsystem1/Subsystem/Frictions ==
  MotorSpeed_radps : Inport
  FrictionCoefficient_Nsprad : Constant  Value=FrictionCoefficient_Nsprad
  Product : Product
  FrictionForce_N : Outport
  wires:
  Product/1 -> FrictionForce_N/1
  MotorSpeed_radps/1 -> Product/2
  FrictionCoefficient_Nsprad/1 -> Product/1

== system comprez/Subsystem3/Subsystem2/AirDrag ==
  VehicleSpeed_mps : Inport
  " " : Constant  Value=0.5
  AirDensity_kgpm3 : Constant  Value=AirDensity_kgpm3
  DragArea_m2 : Constant  Value=DragArea_m2
  DragCoeficient_1 : Constant  Value=DragCoeficient_1
  Product : Product  Inputs=5
  Square : Math  Operator=square  SaturateOnIntegerOverflow=on
  AirDragForce_N : Outport
  wires:
  VehicleSpeed_mps/1 -> Square/1
  Square/1 -> Product/5
  DragArea_m2/1 -> Product/3
  AirDensity_kgpm3/1 -> Product/4
  DragCoeficient_1/1 -> Product/2
  " "/1 -> Product/1
  Product/1 -> AirDragForce_N/1

== system comprez/Subsystem3/Subsystem2/Battery ==
  BatteryCurrent_A : Inport
  1-D Lookup Table : Lookup_n-D  NumberOfTableDimensions=1  BreakpointsForDimension1=BatteryVoltageCoefficient_x  Table=BatteryVoltageCoefficient_y  InternalRulePriority=Speed  RndMeth=Simplest  InputSameDT=on
  BatteryCapacity_Wh : Constant  Value=BatteryCapacity_Wh
  BatteryMaxVoltage_V : Constant  Value=BatteryMaxVoltage_V
  Gain : Gain  Gain=-1
  Gain1 : Gain  Gain=1/3600
  Integrator : Integrator  InitialCondition=BatteryInitialEnergy
  Product : Product
  Product1 : Product  Inputs=*/
  Product2 : Product
  BatteryVoltage_V : Outport
  tag scope: VoltageCoeff=global
  wires:
  BatteryCurrent_A/1 -> Product2/1  "BatteryCurrent_A"
  Product/1 -> Product2/2, BatteryVoltage_V/1  "BatteryVoltage_V"
  Integrator/1 -> Product1/1  "Energy_Wh"
  1-D Lookup Table/1 -> [VoltageCoeff], Product/2  "VoltageCoeficient_0_1"
  BatteryMaxVoltage_V/1 -> Product/1
  BatteryCapacity_Wh/1 -> Product1/2
  Product1/1 -> 1-D Lookup Table/1  "StateOfCharge_0_1"
  Product2/1 -> Gain/1
  Gain/1 -> Gain1/1
  Gain1/1 -> Integrator/1

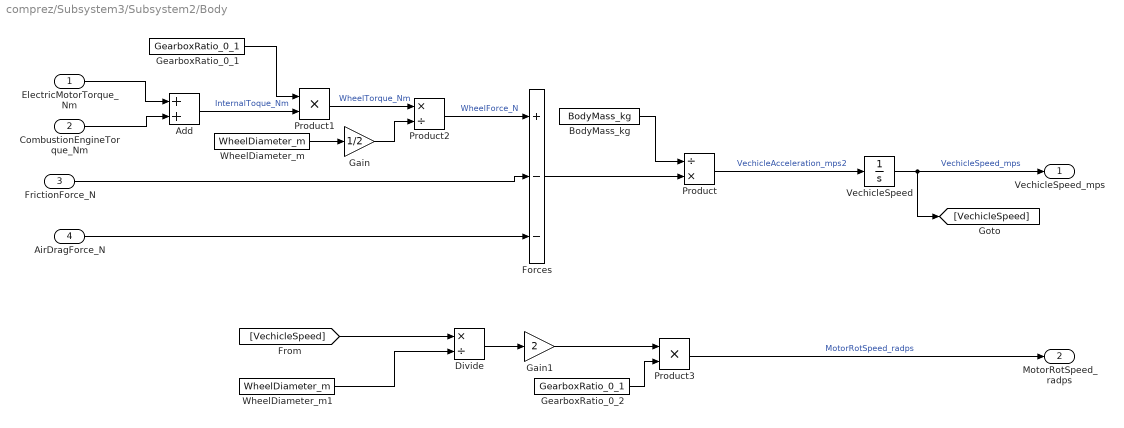
== system comprez/Subsystem3/Subsystem2/Body ==
  ElectricMotorTorque_Nm : Inport
  CombustionEngineTorque_Nm : Inport  Port=2
  FrictionForce_N : Inport  Port=3
  AirDragForce_N : Inport  Port=4
  Add : Sum
  BodyMass_kg : Constant  Value=BodyMass_kg
  Divide : Product  Inputs=*/
  Forces : Sum  Inputs=+--
  Gain : Gain  Gain=1/2
  Gain1 : Gain  Gain=2
  GearboxRatio_0_1 : Constant  Value=GearboxRatio_0_1
  GearboxRatio_0_2 : Constant  Value=GearboxRatio_0_1
  Product : Product  Inputs=/*
  Product1 : Product
  Product2 : Product  Inputs=*/
  Product3 : Product  Inputs=**
  VechicleSpeed : Integrator  InitialCondition=BodyInitialSpeed_mps
  WheelDiameter_m : Constant  Value=WheelDiameter_m
  WheelDiameter_m1 : Constant  Value=WheelDiameter_m
  VechicleSpeed_mps : Outport
  MotorRotSpeed_radps : Outport  Port=2
  wires:
  VechicleSpeed/1 -> [VechicleSpeed], VechicleSpeed_mps/1  "VechicleSpeed_mps"
  Product/1 -> VechicleSpeed/1  "VechicleAcceleration_mps2"
  BodyMass_kg/1 -> Product/1
  Forces/1 -> Product/2
  AirDragForce_N/1 -> Forces/3
  FrictionForce_N/1 -> Forces/2
  ElectricMotorTorque_Nm/1 -> Add/1
  CombustionEngineTorque_Nm/1 -> Add/2
  Add/1 -> Product1/2  "InternalToque_Nm"
  GearboxRatio_0_1/1 -> Product1/1
  Product1/1 -> Product2/1  "WheelTorque_Nm"
  WheelDiameter_m/1 -> Gain/1
  Product2/1 -> Forces/1  "WheelForce_N"
  Gain/1 -> Product2/2
  [VechicleSpeed] -> Divide/1
  WheelDiameter_m1/1 -> Divide/2
  Divide/1 -> Gain1/1
  Gain1/1 -> Product3/1
  GearboxRatio_0_2/1 -> Product3/2
  Product3/1 -> MotorRotSpeed_radps/1  "MotorRotSpeed_radps"

== system comprez/Subsystem3/Subsystem2/CombustionEngine ==
  CombustionEngineStart_1 : Inport
  Gain : Gain  Gain=CombustionEngineMaxTorque_Nm
  Transfer Fcn : TransferFcn  Denominator=[1 1]
  CombustionEngineTorque_Nm : Outport
  wires:
  Transfer Fcn/1 -> CombustionEngineTorque_Nm/1
  CombustionEngineStart_1/1 -> Gain/1
  Gain/1 -> Transfer Fcn/1

== system comprez/Subsystem3/Subsystem2/Driver ==
  BatteryVoltage_V : Inport
  DutyCycle_1 : Inport  Port=2
  Direction_1 : Inport  Port=3
  MotorCurrent_A : Inport  Port=4
  Product : Product
  Product1 : Product
  Product2 : Product
  MotorVoltage_V : Outport
  BatteryCurrent_A : Outport  Port=2
  wires:
  BatteryVoltage_V/1 -> Product/1
  Product/1 -> MotorVoltage_V/1
  Product2/1 -> Product1/1, Product/2
  MotorCurrent_A/1 -> Product1/2
  Product1/1 -> BatteryCurrent_A/1
  DutyCycle_1/1 -> Product2/1
  Direction_1/1 -> Product2/2

== system comprez/Subsystem3/Subsystem2/ElectricMotor ==
  MotorRotSpeed_radps : Inport
  MotorVoltage_V : Inport  Port=2
  Add : Sum  Inputs=-+-
  Constant : Constant  Value=Kt
  Constant1 : Constant  Value=L
  Constant2 : Constant  Value=R
  Constant3 : Constant  Value=Ke
  Integrator : Integrator
  Product : Product
  Product1 : Product  Inputs=*/
  Product2 : Product
  Product3 : Product
  Scope : Scope
  MotorTorque_Nm : Outport
  MotorCurrent_A : Outport  Port=2
  wires:
  Product/1 -> MotorTorque_Nm/1
  Integrator/1 -> MotorCurrent_A/1, Product2/2, Scope/1, Product/2  "MotorCurrent_A"
  Constant/1 -> Product/1
  Product1/1 -> Integrator/1
  Constant1/1 -> Product1/2
  Add/1 -> Product1/1
  Product2/1 -> Add/3
  Constant2/1 -> Product2/1
  MotorVoltage_V/1 -> Add/2
  Constant3/1 -> Product3/1
  Product3/1 -> Add/1
  MotorRotSpeed_radps/1 -> Product3/2

== system comprez/Subsystem3/Subsystem2/Frictions ==
  MotorSpeed_radps : Inport
  FrictionCoefficient_Nsprad : Constant  Value=FrictionCoefficient_Nsprad
  Product : Product
  FrictionForce_N : Outport
  wires:
  Product/1 -> FrictionForce_N/1
  MotorSpeed_radps/1 -> Product/2
  FrictionCoefficient_Nsprad/1 -> Product/1

== matlab function comprez/Subsystem/MATLAB Function ==
  data: e input; s output; eq input; lambda input
function s = fcn(e,eq,lambda)

s = lambda*e + eq;

end
